simulink model "SVPWM1_LD"  (Simulink 10.1)
settings: Solver=ode45  StartTime=0.0  StopTime=0.2  RelTol=1e-3  EnableMultiTasking=on
libraries: powerlib x20, powerlib_extras x3, simulink x2
settings Model: Creator=Administrator  LastModifiedBy=ZhuanZ（无密码）
settings DataIOCC: LimitDataPoints=on  SignalLoggingSaveFormat=ModelDataLogs
settings OptimizationCC: ExpressionDepthLimit=2147483647
settings DebuggingCC: SolverPrmCheckMsg=warning  FcnCallInpInsideContextMsg=warning  StateNameClashWarn=warning
settings SFSimCC: SimParseCustomCode=off
settings SimscapeCC: SimscapeNormalizeSystem=off

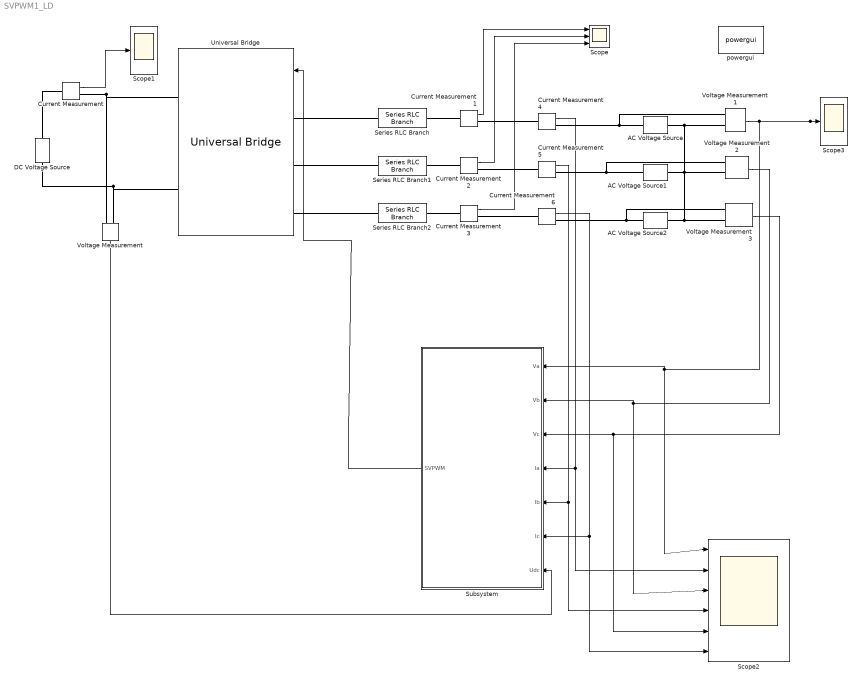
== system SVPWM1_LD ==
  AC Voltage Source : powerlib/Electrical Sources/AC Voltage Source  Amplitude=380  Phase=90  Frequency=50  SampleTime=0  Measurements=None  BusType=swing  Pref=10e3  Qref=0  Qmin=-inf  Qmax=+inf
  AC Voltage Source1 : powerlib/Electrical Sources/AC Voltage Source  Amplitude=380  Phase=90-120  Frequency=50  SampleTime=0  Measurements=None  BusType=swing  Pref=10e3  Qref=0  Qmin=-inf  Qmax=+inf
  AC Voltage Source2 : powerlib/Electrical Sources/AC Voltage Source  Amplitude=380  Phase=90+120  Frequency=50  SampleTime=0  Measurements=None  BusType=swing  Pref=10e3  Qref=0  Qmin=-inf  Qmax=+inf
  Current Measurement{,1..6} (7 alike) : powerlib/Measurements/Current Measurement  PhasorSimulation=off  OutputType=Complex  PSBequivalent=0
  DC Voltage Source : powerlib/Electrical Sources/DC Voltage Source  Amplitude=100  Measurements=None
  Scope : Scope  NumInputPorts=3
  Scope1 : Scope
  Scope2 : Scope  NumInputPorts=6
  Scope3 : Scope
  Series RLC Branch : powerlib/Elements/Series RLC Branch  LConnTagsString=__new0  RConnTagsString=__new0  BranchType=RL  Resistance=1  Inductance=6e-3  SetiL0=off  InitialCurrent=0  Capacitance=1.0  Setx0=off  InitialVoltage=0  Measurements=None
  Series RLC Branch1 : powerlib/Elements/Series RLC Branch  LConnTagsString=__new0  RConnTagsString=__new0  BranchType=RL  Resistance=1  Inductance=6e-3  SetiL0=off  InitialCurrent=0  Capacitance=1.0  Setx0=off  InitialVoltage=0  Measurements=None
  Series RLC Branch2 : powerlib/Elements/Series RLC Branch  LConnTagsString=__new0  RConnTagsString=__new0  BranchType=RL  Resistance=1  Inductance=6e-3  SetiL0=off  InitialCurrent=0  Capacitance=1.0  Setx0=off  InitialVoltage=0  Measurements=None
  Subsystem : Subsystem
  Universal Bridge : powerlib/Power Electronics/Universal Bridge  Arms=3  SnubberResistance=1e5  SnubberCapacitance=inf  Device=Thyristors  Ron=1e-3  Lon=0  ForwardVoltages="[  0  0  ]"  ForwardVoltage=0  GTOparameters=[ 10e-6 , 20e-6 ]  IGBTparameters=[ 1e-6 , 2e-6 ]  Measurements=None  Measurements_2=None  converterType=Rectifier
  Voltage Measurement{,1..3} (4 alike) : powerlib/Measurements/Voltage Measurement  PhasorSimulation=off  OutputType=Complex  PSBequivalent=0
  powergui : powerlib/powergui  Priority=1  SimulationMode=Continuous  SampleTime=50e-6  frequency=60  Iterations=50  frequencyindice=50  Pbase=100e6  ErrMax=1e-4  UnitsV=kV  UnitsW=MW  buscounter=0  FunctionMessages=off  echomessages=off  EnableUseOfTLC=off  CurrentSourceSwitches=off  DisableSnubberDevices=off  DisableRonSwitches=off  DisableVfSwitches=off  DisplayEquations=off  AutomaticDiscreteSolvers=off  SolverType=Tustin/Backward Euler (TBE)  Interpol=off  ExternalGateDelay=off  methode=off  Ts=0  x0status=blocks  SPID=off  SwTol=0  HookPort=off  NonlinearTolerance=1e-4  nMaxIteration=100  ContinueOnMaxIteration=off  RestoreLinks=warning  ResistiveCurrentMeasurement=off  Frange=[0:2:500]  Ylog=off  Xlog=on  ShowGrid=off  save=off  variable=ZData  structure=0  ZoomFFT=on  StartTime=0.0  cycles=1  DisplayStyle=1  fundamental=60  FreqAxis=off  MaxFrequency=1000  frequencyindicesteady=1  RmsSteady=1  display=off
  wires:
  Current Measurement1/1 -> Scope/1
  Current Measurement2/1 -> Scope/2
  Current Measurement3/1 -> Scope/3
  Voltage Measurement/1 -> Subsystem/7(Udc)
  Voltage Measurement1/1 -> Subsystem/1(Va), Scope2/1, Scope3/1
  Voltage Measurement2/1 -> Subsystem/2(Vb), Scope2/3
  Voltage Measurement3/1 -> Subsystem/3(Vc), Scope2/5
  Current Measurement4/1 -> Subsystem/4(Ia), Scope2/2
  Current Measurement5/1 -> Subsystem/5(Ib), Scope2/4
  Current Measurement6/1 -> Subsystem/6(Ic), Scope2/6
  Current Measurement/1 -> Scope1/1
  Subsystem/1(SVPWM) -> Universal Bridge/1
  connections:
  DC Voltage Source/RConn1 -- Current Measurement/LConn1
  Current Measurement/RConn1 -- Universal Bridge/RConn1 -- Voltage Measurement/LConn1
  DC Voltage Source/LConn1 -- Universal Bridge/RConn2 -- Voltage Measurement/LConn2
  Universal Bridge/LConn1 -- Series RLC Branch/LConn1
  Universal Bridge/LConn2 -- Series RLC Branch1/LConn1
  Universal Bridge/LConn3 -- Series RLC Branch2/LConn1
  Series RLC Branch/RConn1 -- Current Measurement1/LConn1
  Series RLC Branch1/RConn1 -- Current Measurement2/LConn1
  Series RLC Branch2/RConn1 -- Current Measurement3/LConn1
  Current Measurement1/RConn1 -- Current Measurement4/LConn1
  Current Measurement2/RConn1 -- Current Measurement5/LConn1
  Current Measurement3/RConn1 -- Current Measurement6/LConn1
  AC Voltage Source/RConn1 -- Current Measurement4/RConn1 -- Voltage Measurement1/LConn1
  AC Voltage Source1/RConn1 -- Current Measurement5/RConn1 -- Voltage Measurement2/LConn1
  AC Voltage Source2/RConn1 -- Current Measurement6/RConn1 -- Voltage Measurement3/LConn1
  AC Voltage Source2/LConn1 -- Voltage Measurement1/LConn2 -- AC Voltage Source/LConn1 -- Voltage Measurement2/LConn2 -- AC Voltage Source1/LConn1 -- Voltage Measurement3/LConn2

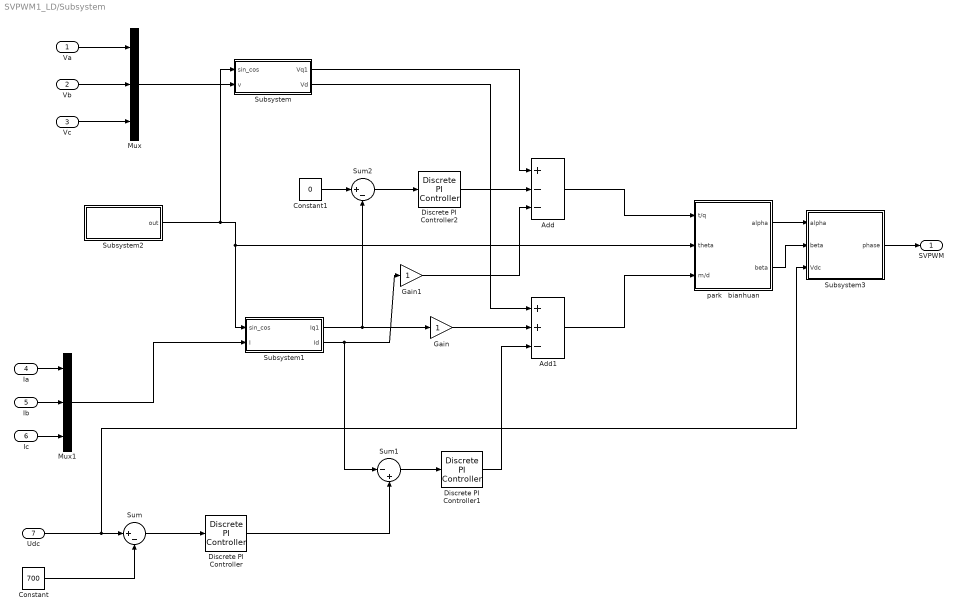
== system SVPWM1_LD/Subsystem ==
  Va : Inport
  Vb : Inport  Port=2
  Vc : Inport  Port=3
  Ia : Inport  Port=4
  Ib : Inport  Port=5
  Ic : Inport  Port=6
  Udc : Inport  Port=7
  Add : Sum  Inputs=+--
  Add1 : Sum  Inputs=++-
  Constant : Constant  Value=700
  Constant1 : Constant  Value=0
  Discrete PI Controller : powerlib_extras/Discrete  Control Blocks/Discrete PI Controller  Kp=0.1  Ki=1  Par_Limits=[1e6 -1e6]  Init=0  Ts=50e-6
  Discrete PI Controller1 : powerlib_extras/Discrete  Control Blocks/Discrete PI Controller  Kp=0.1  Ki=1  Par_Limits=[1e6 -1e6]  Init=0  Ts=50e-6
  Discrete PI Controller2 : powerlib_extras/Discrete  Control Blocks/Discrete PI Controller  Kp=0.1  Ki=1  Par_Limits=[1e6 -1e6]  Init=0  Ts=50e-6
  Gain : Gain
  Gain1 : Gain
  Mux : Mux  Inputs=3
  Mux1 : Mux  Inputs=3
  Subsystem : Subsystem
  Subsystem1 : Subsystem
  Subsystem2 : Subsystem
  Subsystem3 : Subsystem
  Sum : Sum  Inputs=|+-
  Sum1 : Sum  Inputs=|-+
  Sum2 : Sum  Inputs=|+-
  park   bianhuan : Subsystem
  SVPWM : Outport
  wires:
  Va/1 -> Mux/1
  Vb/1 -> Mux/2
  Vc/1 -> Mux/3
  Mux/1 -> Subsystem/2(v)
  Subsystem2/1(out) -> Subsystem/1(sin_cos), park   bianhuan/2(theta), Subsystem1/1(sin_cos)
  Ia/1 -> Mux1/1
  Ib/1 -> Mux1/2
  Ic/1 -> Mux1/3
  Mux1/1 -> Subsystem1/2(I)
  Udc/1 -> Sum/1, Subsystem3/3(Vdc)
  Constant/1 -> Sum/2
  Sum/1 -> Discrete PI Controller/1
  Discrete PI Controller/1 -> Sum1/2
  Subsystem1/2(Id) -> Sum1/1, Gain1/1
  Subsystem1/1(Iq1) -> Gain/1, Sum2/2
  Sum1/1 -> Discrete PI Controller1/1
  Constant1/1 -> Sum2/1
  Sum2/1 -> Discrete PI Controller2/1
  Discrete PI Controller2/1 -> Add/2
  Subsystem/1(Vq1) -> Add/1
  Subsystem/2(Vd) -> Add1/1
  Gain1/1 -> Add/3
  Gain/1 -> Add1/2
  Discrete PI Controller1/1 -> Add1/3
  Add/1 -> park   bianhuan/1(t/q)
  Add1/1 -> park   bianhuan/3(m/d)
  park   bianhuan/1(alpha) -> Subsystem3/1(alpha)
  park   bianhuan/2(beta) -> Subsystem3/2(beta)
  Subsystem3/1(phase) -> SVPWM/1

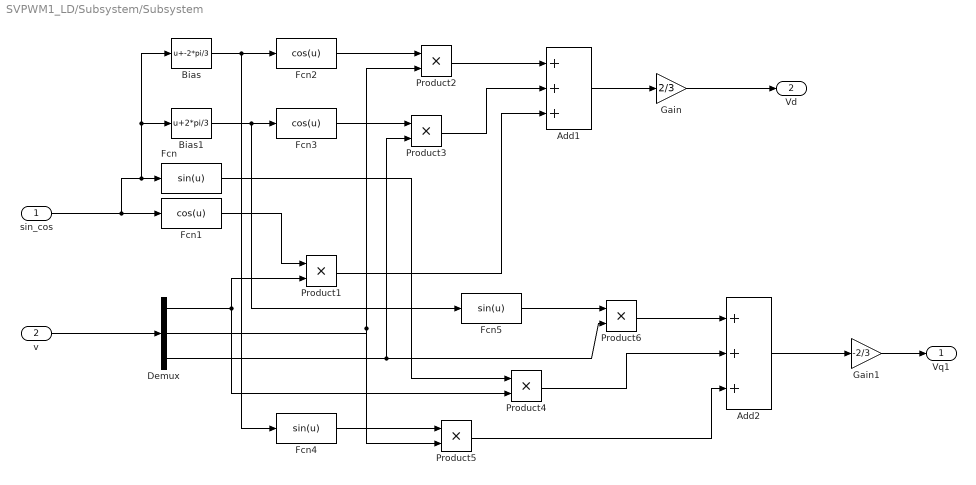
== system SVPWM1_LD/Subsystem/Subsystem ==
  sin_cos : Inport
  v : Inport  Port=2
  Add1 : Sum  Inputs=+++
  Add2 : Sum  Inputs=+++
  Bias : Bias  Bias=-2*pi/3
  Bias1 : Bias  Bias=2*pi/3
  Demux : Demux  Outputs=3
  Fcn : Fcn  Expr=sin(u)
  Fcn1 : Fcn  Expr=cos(u)
  Fcn2 : Fcn  Expr=cos(u)
  Fcn3 : Fcn  Expr=cos(u)
  Fcn4 : Fcn  Expr=sin(u)
  Fcn5 : Fcn  Expr=sin(u)
  Gain : Gain  Gain=2/3
  Gain1 : Gain  Gain=-2/3
  Product{1..6} (6 alike) : Product  RndMeth=Zero
  Vq1 : Outport
  Vd : Outport  Port=2
  wires:
  v/1 -> Demux/1
  Demux/1 -> Product1/2, Product4/2
  Fcn1/1 -> Product1/1
  Bias/1 -> Fcn2/1, Fcn4/1
  Demux/2 -> Product2/2, Product5/2
  Fcn2/1 -> Product2/1
  Bias1/1 -> Fcn3/1, Fcn5/1
  Fcn3/1 -> Product3/1
  Demux/3 -> Product3/2, Product6/2
  Product2/1 -> Add1/1
  Product3/1 -> Add1/2
  Product1/1 -> Add1/3
  Add1/1 -> Gain/1
  Gain/1 -> Vd/1
  Fcn/1 -> Product4/1
  Fcn4/1 -> Product5/1
  Fcn5/1 -> Product6/1
  Product6/1 -> Add2/1
  Product4/1 -> Add2/2
  Product5/1 -> Add2/3
  Add2/1 -> Gain1/1
  Gain1/1 -> Vq1/1
  sin_cos/1 -> Fcn1/1, Fcn/1, Bias/1, Bias1/1

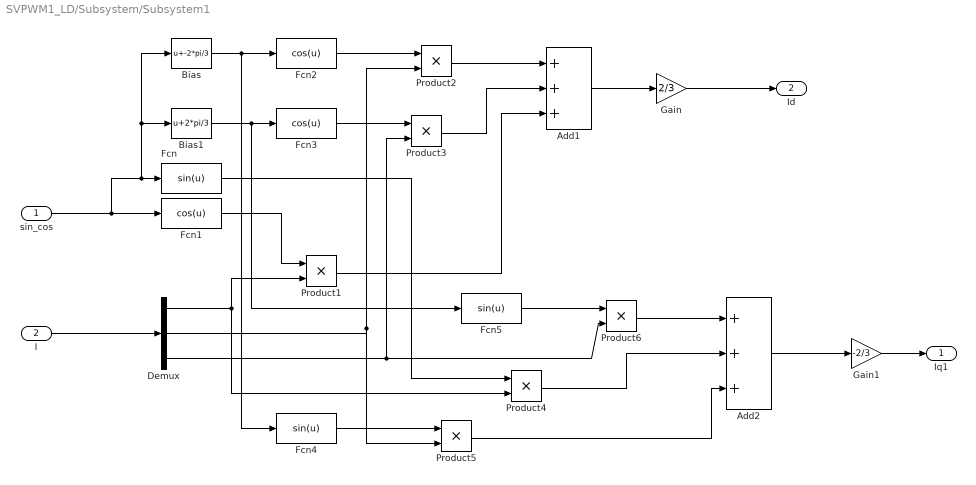
== system SVPWM1_LD/Subsystem/Subsystem1 ==
  sin_cos : Inport
  I : Inport  Port=2
  Add1 : Sum  Inputs=+++
  Add2 : Sum  Inputs=+++
  Bias : Bias  Bias=-2*pi/3
  Bias1 : Bias  Bias=2*pi/3
  Demux : Demux  Outputs=3
  Fcn : Fcn  Expr=sin(u)
  Fcn1 : Fcn  Expr=cos(u)
  Fcn2 : Fcn  Expr=cos(u)
  Fcn3 : Fcn  Expr=cos(u)
  Fcn4 : Fcn  Expr=sin(u)
  Fcn5 : Fcn  Expr=sin(u)
  Gain : Gain  Gain=2/3
  Gain1 : Gain  Gain=-2/3
  Product{1..6} (6 alike) : Product  RndMeth=Zero
  Iq1 : Outport
  Id : Outport  Port=2
  wires:
  I/1 -> Demux/1
  sin_cos/1 -> Fcn1/1, Fcn/1, Bias/1, Bias1/1
  Demux/1 -> Product1/2, Product4/2
  Fcn1/1 -> Product1/1
  Bias/1 -> Fcn2/1, Fcn4/1
  Demux/2 -> Product2/2, Product5/2
  Fcn2/1 -> Product2/1
  Bias1/1 -> Fcn3/1, Fcn5/1
  Fcn3/1 -> Product3/1
  Demux/3 -> Product3/2, Product6/2
  Product2/1 -> Add1/1
  Product3/1 -> Add1/2
  Product1/1 -> Add1/3
  Add1/1 -> Gain/1
  Gain/1 -> Id/1
  Fcn/1 -> Product4/1
  Fcn4/1 -> Product5/1
  Fcn5/1 -> Product6/1
  Product6/1 -> Add2/1
  Product4/1 -> Add2/2
  Product5/1 -> Add2/3
  Add2/1 -> Gain1/1
  Gain1/1 -> Iq1/1

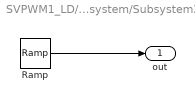
== system SVPWM1_LD/Subsystem/Subsystem2 ==
  Ramp : simulink/Sources/Ramp  slope=100*pi  start=0  InitialOutput=0
  out : Outport
  wires:
  Ramp/1 -> out/1

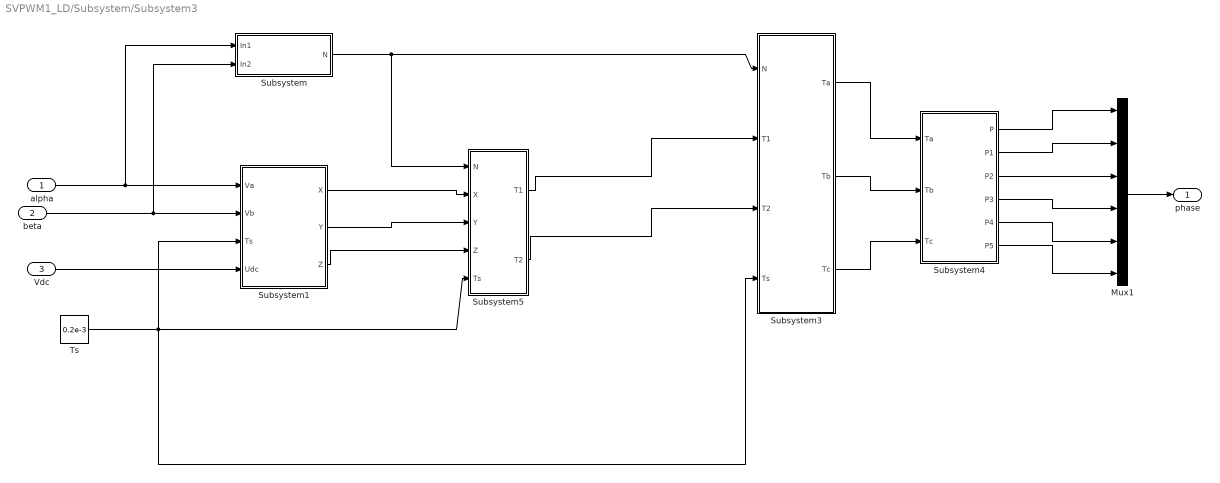
== system SVPWM1_LD/Subsystem/Subsystem3 ==
  alpha : Inport
  beta : Inport  Port=2
  Vdc : Inport  Port=3
  Mux1 : Mux  Inputs=6
  Subsystem : Subsystem
  Subsystem1 : Subsystem
  Subsystem3 : Subsystem
  Subsystem4 : Subsystem
  Subsystem5 : Subsystem
  Ts : Constant  Value=0.2e-3
  phase : Outport
  wires:
  alpha/1 -> Subsystem1/1(Va), Subsystem/1(In1)
  beta/1 -> Subsystem1/2(Vb), Subsystem/2(In2)
  Ts/1 -> Subsystem1/3(Ts), Subsystem5/5(Ts), Subsystem3/4(Ts)
  Subsystem4/1(P) -> Mux1/1
  Subsystem4/2(P1) -> Mux1/2
  Subsystem4/3(P2) -> Mux1/3
  Subsystem4/4(P3) -> Mux1/4
  Subsystem4/5(P4) -> Mux1/5
  Subsystem4/6(P5) -> Mux1/6
  Subsystem/1(N) -> Subsystem5/1(N), Subsystem3/1(N)
  Subsystem1/1(X) -> Subsystem5/2(X)
  Subsystem1/2(Y) -> Subsystem5/3(Y)
  Subsystem1/3(Z) -> Subsystem5/4(Z)
  Subsystem5/1(T1) -> Subsystem3/2(T1)
  Subsystem5/2(T2) -> Subsystem3/3(T2)
  Vdc/1 -> Subsystem1/4(Udc)
  Subsystem3/1(Ta) -> Subsystem4/1(Ta)
  Subsystem3/2(Tb) -> Subsystem4/2(Tb)
  Subsystem3/3(Tc) -> Subsystem4/3(Tc)
  Mux1/1 -> phase/1

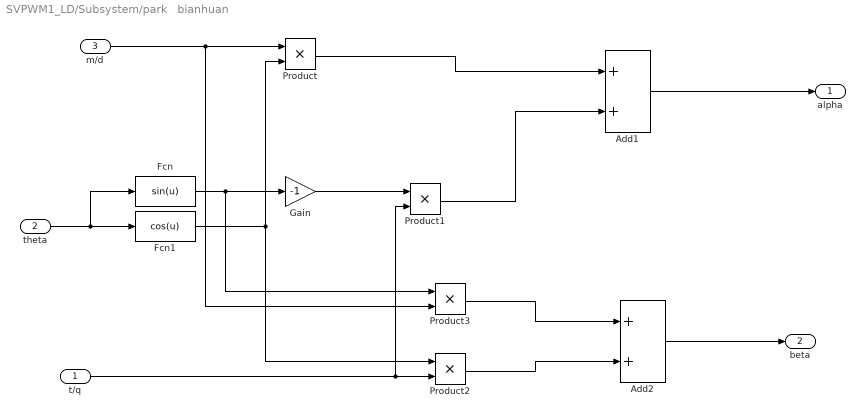
== system SVPWM1_LD/Subsystem/park   bianhuan ==
  t/q : Inport
  theta : Inport  Port=2
  m/d : Inport  Port=3
  Add1 : Sum
  Add2 : Sum
  Fcn : Fcn  Expr=sin(u)
  Fcn1 : Fcn  Expr=cos(u)
  Gain : Gain  Gain=-1
  Product{,1..3} (4 alike) : Product  RndMeth=Zero
  alpha : Outport
  beta : Outport  Port=2
  wires:
  theta/1 -> Fcn1/1, Fcn/1
  m/d/1 -> Product/1, Product3/2
  t/q/1 -> Product1/2, Product2/2
  Gain/1 -> Product1/1
  Fcn/1 -> Gain/1, Product3/1
  Fcn1/1 -> Product/2, Product2/1
  Product/1 -> Add1/1
  Product1/1 -> Add1/2
  Product3/1 -> Add2/1
  Product2/1 -> Add2/2
  Add2/1 -> beta/1
  Add1/1 -> alpha/1

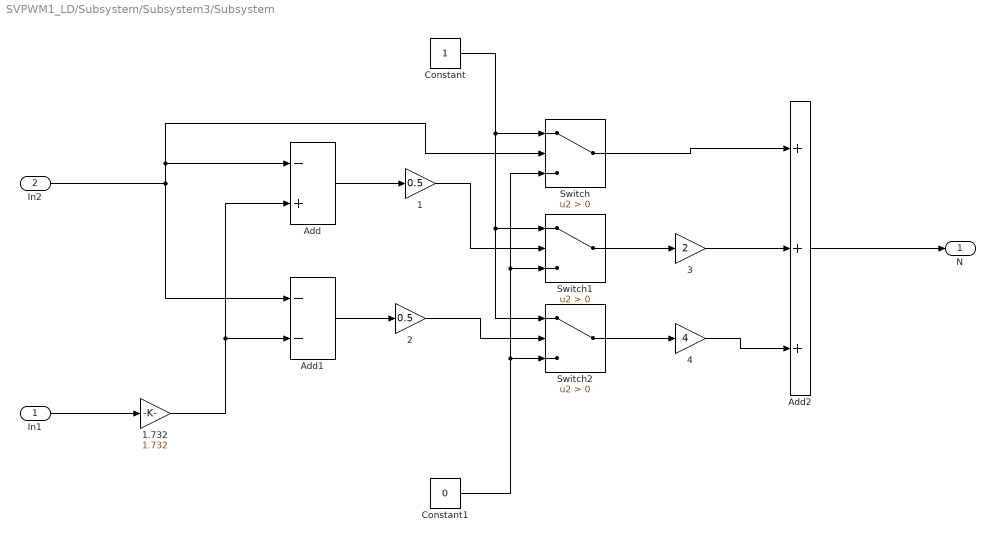
== system SVPWM1_LD/Subsystem/Subsystem3/Subsystem ==
  In1 : Inport
  In2 : Inport  Port=2
  1 : Gain  Gain=0.5
  1.732 : Gain  Gain=1.732
  2 : Gain  Gain=0.5
  3 : Gain  Gain=2
  4 : Gain  Gain=4
  Add : Sum  Inputs=-+
  Add1 : Sum  Inputs=--
  Add2 : Sum  Inputs=+++
  Constant : Constant
  Constant1 : Constant  Value=0
  Switch : Switch  Criteria=u2 > Threshold
  Switch1 : Switch  Criteria=u2 > Threshold
  Switch2 : Switch  Criteria=u2 > Threshold
  N : Outport
  wires:
  In2/1 -> Add1/1, Add/1, Switch/2
  1.732/1 -> Add1/2, Add/2
  In1/1 -> 1.732/1
  Add1/1 -> 2/1
  Add/1 -> 1/1
  1/1 -> Switch1/2
  2/1 -> Switch2/2
  Constant/1 -> Switch/1, Switch1/1, Switch2/1
  Constant1/1 -> Switch2/3, Switch1/3, Switch/3
  Switch1/1 -> 3/1
  Switch2/1 -> 4/1
  Switch/1 -> Add2/1
  3/1 -> Add2/2
  4/1 -> Add2/3
  Add2/1 -> N/1

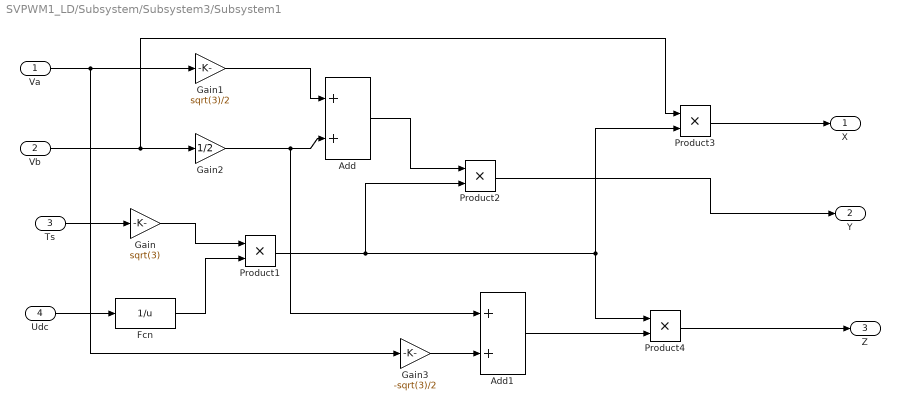
== system SVPWM1_LD/Subsystem/Subsystem3/Subsystem1 ==
  Va : Inport
  Vb : Inport  Port=2
  Ts : Inport  Port=3
  Udc : Inport  Port=4
  Add : Sum
  Add1 : Sum
  Fcn : Fcn  Expr=1/u
  Gain : Gain  Gain=sqrt(3)
  Gain1 : Gain  Gain=sqrt(3)/2
  Gain2 : Gain  Gain=1/2
  Gain3 : Gain  Gain=-sqrt(3)/2
  Product{1..4} (4 alike) : Product  RndMeth=Zero
  X : Outport
  Y : Outport  Port=2
  Z : Outport  Port=3
  wires:
  Udc/1 -> Fcn/1
  Ts/1 -> Gain/1
  Gain/1 -> Product1/1
  Fcn/1 -> Product1/2
  Va/1 -> Gain1/1, Gain3/1
  Vb/1 -> Gain2/1, Product3/1
  Gain1/1 -> Add/1
  Gain2/1 -> Add/2, Add1/1
  Add/1 -> Product2/1
  Product1/1 -> Product2/2, Product3/2, Product4/1
  Product2/1 -> Y/1
  Product3/1 -> X/1
  Gain3/1 -> Add1/2
  Add1/1 -> Product4/2
  Product4/1 -> Z/1

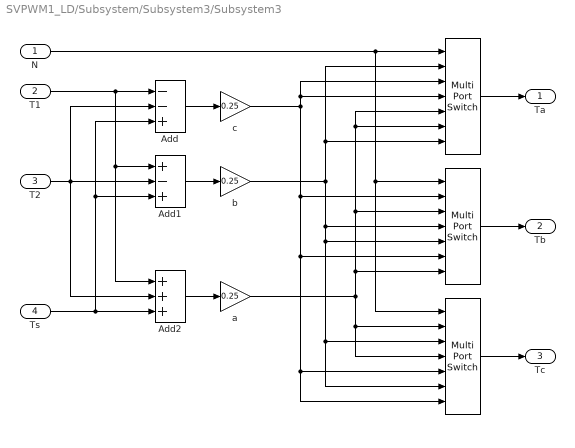
== system SVPWM1_LD/Subsystem/Subsystem3/Subsystem3 ==
  N : Inport
  T1 : Inport  Port=2
  T2 : Inport  Port=3
  Ts : Inport  Port=4
  " " : MultiPortSwitch  Inputs=6
  "  " : MultiPortSwitch  Inputs=6
  "    " : MultiPortSwitch  Inputs=6
  Add : Sum  Inputs=--+
  Add1 : Sum  Inputs=+-+
  Add2 : Sum  Inputs=+++
  a : Gain  Gain=0.25
  b : Gain  Gain=0.25
  c : Gain  Gain=0.25
  Ta : Outport
  Tb : Outport  Port=2
  Tc : Outport  Port=3
  wires:
  N/1 -> "  "/1, " "/1, "    "/1
  T1/1 -> Add/1, Add1/1, Add2/1
  T2/1 -> Add/2, Add1/2, Add2/2
  Ts/1 -> Add/3, Add1/3, Add2/3
  Add/1 -> c/1
  Add1/1 -> b/1
  Add2/1 -> a/1
  "  "/1 -> Ta/1
  " "/1 -> Tb/1
  "    "/1 -> Tc/1
  b/1 -> "  "/7, "  "/2, " "/4, " "/5, "    "/3, "    "/6
  c/1 -> " "/2, " "/6, "    "/5, "    "/7, "  "/4, "  "/3
  a/1 -> "  "/5, "  "/6, " "/3, " "/7, "    "/2, "    "/4

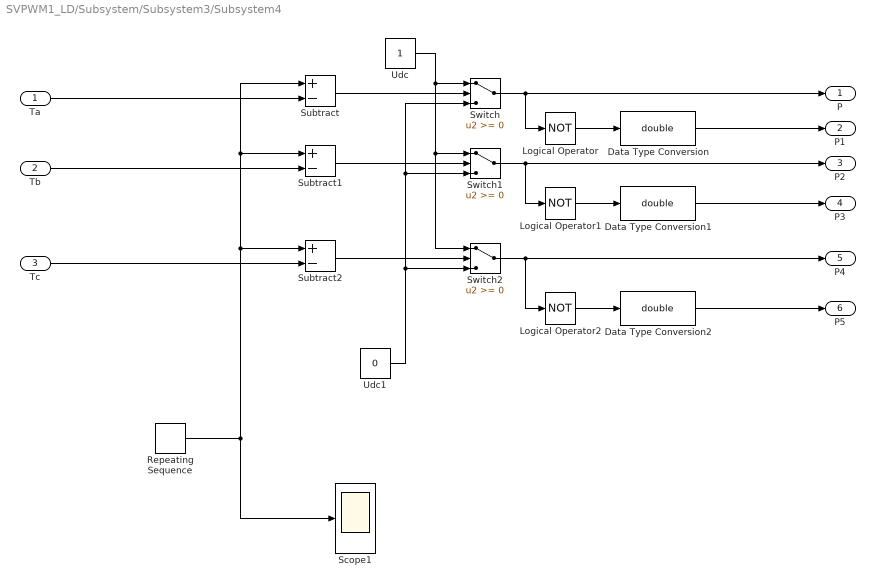
== system SVPWM1_LD/Subsystem/Subsystem3/Subsystem4 ==
  Ta : Inport
  Tb : Inport  Port=2
  Tc : Inport  Port=3
  Data Type Conversion : DataTypeConversion  OutDataTypeStr=double
  Data Type Conversion1 : DataTypeConversion  OutDataTypeStr=double
  Data Type Conversion2 : DataTypeConversion  OutDataTypeStr=double
  Logical Operator : Logic  Operator=NOT  AllPortsSameDT=off  OutDataTypeStr=boolean
  Logical Operator1 : Logic  Operator=NOT  AllPortsSameDT=off  OutDataTypeStr=boolean
  Logical Operator2 : Logic  Operator=NOT  AllPortsSameDT=off  OutDataTypeStr=boolean
  Repeating Sequence : simulink/Sources/Repeating Sequence  rep_seq_t="[0  1e-4  2e-4]"  rep_seq_y="[0  1e-4   0]"
  Scope1 : Scope
  Subtract : Sum  Inputs=+-
  Subtract1 : Sum  Inputs=+-
  Subtract2 : Sum  Inputs=+-
  Switch : Switch
  Switch1 : Switch
  Switch2 : Switch
  Udc : Constant
  Udc1 : Constant  Value=0
  P : Outport
  P1 : Outport  Port=2
  P2 : Outport  Port=3
  P3 : Outport  Port=4
  P4 : Outport  Port=5
  P5 : Outport  Port=6
  wires:
  Repeating Sequence/1 -> Subtract/1, Subtract1/1, Subtract2/1, Scope1/1
  Subtract2/1 -> Switch2/2
  Subtract1/1 -> Switch1/2
  Subtract/1 -> Switch/2
  Udc/1 -> Switch/1, Switch1/1, Switch2/1
  Udc1/1 -> Switch2/3, Switch1/3, Switch/3
  Switch/1 -> P/1, Logical Operator/1
  Switch1/1 -> P2/1, Logical Operator1/1
  Switch2/1 -> P4/1, Logical Operator2/1
  Logical Operator/1 -> Data Type Conversion/1
  Data Type Conversion/1 -> P1/1
  Logical Operator1/1 -> Data Type Conversion1/1
  Data Type Conversion1/1 -> P3/1
  Logical Operator2/1 -> Data Type Conversion2/1
  Data Type Conversion2/1 -> P5/1
  Ta/1 -> Subtract/2
  Tb/1 -> Subtract1/2
  Tc/1 -> Subtract2/2

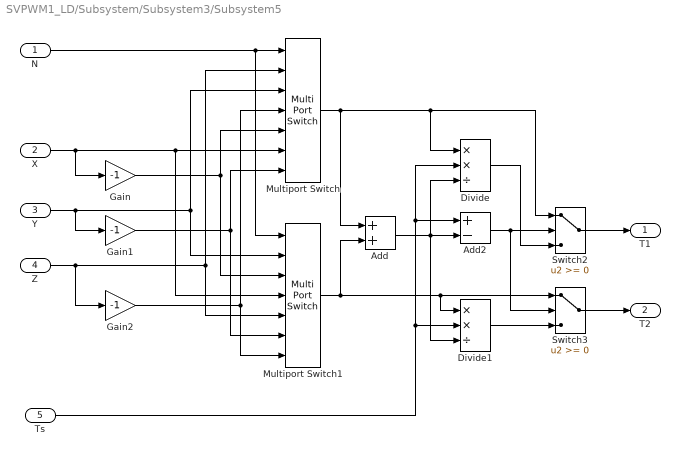
== system SVPWM1_LD/Subsystem/Subsystem3/Subsystem5 ==
  N : Inport
  X : Inport  Port=2
  Y : Inport  Port=3
  Z : Inport  Port=4
  Ts : Inport  Port=5
  Add : Sum
  Add2 : Sum  Inputs=+-
  Divide : Product  Inputs=**/
  Divide1 : Product  Inputs=**/
  Gain : Gain  Gain=-1
  Gain1 : Gain  Gain=-1
  Gain2 : Gain  Gain=-1
  Multiport Switch : MultiPortSwitch  Inputs=6
  Multiport Switch1 : MultiPortSwitch  Inputs=6
  Switch2 : Switch
  Switch3 : Switch
  T1 : Outport
  T2 : Outport  Port=2
  wires:
  N/1 -> Multiport Switch/1, Multiport Switch1/1
  Multiport Switch/1 -> Add/1, Divide/1, Switch2/1
  Multiport Switch1/1 -> Add/2, Switch3/1, Divide1/1
  Ts/1 -> Divide1/2, Divide/2, Add2/1
  Add2/1 -> Switch2/2, Switch3/2
  Divide/1 -> Switch2/3
  Divide1/1 -> Switch3/3
  Switch3/1 -> T2/1
  Switch2/1 -> T1/1
  Add/1 -> Divide/3, Divide1/3, Add2/2
  Gain1/1 -> Multiport Switch1/6, Multiport Switch/7
  Gain2/1 -> Multiport Switch/4, Multiport Switch1/7
  Gain/1 -> Multiport Switch/5, Multiport Switch1/3
  Y/1 -> Gain1/1, Multiport Switch/3, Multiport Switch1/2
  X/1 -> Gain/1, Multiport Switch/6, Multiport Switch1/4
  Z/1 -> Gain2/1, Multiport Switch/2, Multiport Switch1/5
